simulink model "AM_passband"  (R2026a)
settings: Solver=VariableStepAuto  StopTime=1
model workspace (MAT data in the model file):
  FrameSize = 1000
  Fs = 100000
libraries: dspsrcs4 x3, dspfdesign x2, commchan3 x1
settings Model: Creator=ranja  LastModifiedBy=ranja

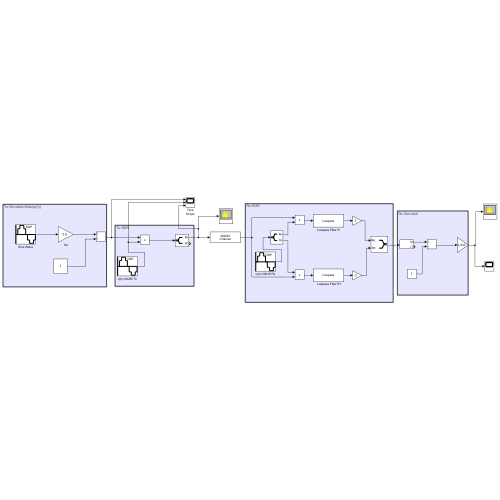
[thumbnail: Simulink's stored preview of the top-level diagram]
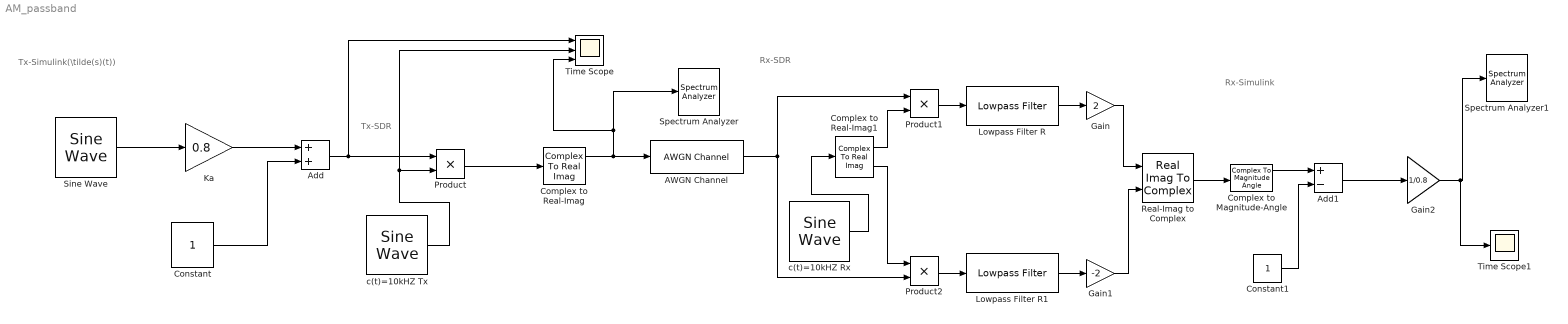
== system AM_passband ==
  note: Rx-Simulink
  note: Rx-SDR
  note: Tx-SDR
  note: Tx-Simulink(\tilde(s)(t))
  " Ka" : Gain  Gain=0.8
  AWGN Channel : commchan3/AWGN Channel  LegacyMode=off  NoiseMethod="Signal to noise ratio  (SNR)"  noiseMode="Signal to noise ratio  (SNR)"  EbNo=10  EsNo=10  SNR=10  BitsPerSymbol=1  SignalPower=1  SpecifySymbolPeriod=off  SamplesPerSymbol=1  SymbolPeriod=1  VarianceSource=Parameter  Variance=1  RandomStream=Global stream  Seed=67  SimulateUsing=Code generation
  Add : Sum
  Add1 : Sum  Inputs=+-
  Complex to Magnitude-Angle : ComplexToMagnitudeAngle
  Complex to Real-Imag : ComplexToRealImag
  Complex to Real-Imag1 : ComplexToRealImag
  Constant : Constant
  Constant1 : Constant
  Gain : Gain  Gain=2
  Gain1 : Gain  Gain=-2
  Gain2 : Gain  Gain=1/0.8
  Lowpass Filter R : dspfdesign/Lowpass Filter  FilterType=FIR  DesignForMinimumOrder=off  FilterOrder=50  PassbandFrequency=1100  StopbandFrequency=0.5442  PassbandRipple=0.1  StopbandAttenuation=80  SampleRateMode=Specify on dialog  SampleRate=Fs  SimulateUsing=Interpreted execution  roundingMode=Floor  coeffsDataTypeStr=fixdt(1,16)
  Lowpass Filter R1 : dspfdesign/Lowpass Filter  FilterType=FIR  DesignForMinimumOrder=off  FilterOrder=50  PassbandFrequency=1100  StopbandFrequency=0.5442  PassbandRipple=0.1  StopbandAttenuation=80  SampleRateMode=Specify on dialog  SampleRate=Fs  SimulateUsing=Interpreted execution  roundingMode=Floor  coeffsDataTypeStr=fixdt(1,16)
  Product : Product
  Product1 : Product
  Product2 : Product
  Real-Imag to Complex : RealImagToComplex
  Sine Wave : dspsrcs4/Sine Wave  Amplitude=1  Frequency=1000  Phase=0  SampleMode=Discrete  OutComplex=Real  CompMethod=Trigonometric fcn  TableSize=Speed  SampleTime=1/Fs  SamplesPerFrame=FrameSize  ResetState=Restart at time zero  OutputFrames=off  dataType=double  wordLen=16  udDataType=sfix(16)  fracBitsMode=Best precision  numFracBits=15  OutDataTypeStr=double  LastOutDataTypeStr=double
  Spectrum Analyzer : SpectrumAnalyzer  WindowPosition=[368.000000,182.000000,800.000000,500.000000,]  ScopeFrameLocation=window  WindowInvariantSamplesPerUpdate=on  Span=100000  StartFrequency=-50000  StopFrequency=50000  YLimits=[-83.7362 34.2546]
  Spectrum Analyzer1 : SpectrumAnalyzer  WindowPosition=[1.000000,49.000000,1536.000000,793.000000,]  ScopeFrameLocation=window  WindowInvariantSamplesPerUpdate=on  FrequencySpan=Span and center frequency  Span=50000  StartFrequency=-50000  StopFrequency=50000  YLimits=[-68.0974 28.8861]  SelectedToolstripTab=spectrumAnalyzerToolstrip.estimationTab
  Time Scope : Scope  NumInputPorts=3
      settings: TimeUnits=Metric (based on Time Span)  ActiveDisplayYMinimum=0.21609485710194476  ActiveDisplayYMaximum=1.7356972505215549  YLabel=Amplitude
  Time Scope1 : Scope
      settings: TimeUnits=Metric (based on Time Span)  ActiveDisplayYMinimum=-1.3427014205665166  ActiveDisplayYMaximum=1.6995374742641378  YLabel=Amplitude
  c(t)=10kHZ Rx : dspsrcs4/Sine Wave  Amplitude=1  Frequency=10000  Phase=0  SampleMode=Discrete  OutComplex=Complex  CompMethod=Trigonometric fcn  TableSize=Speed  SampleTime=1/Fs  SamplesPerFrame=FrameSize  ResetState=Restart at time zero  OutputFrames=off  dataType=double  wordLen=16  udDataType=sfix(16)  fracBitsMode=Best precision  numFracBits=15  OutDataTypeStr=double  LastOutDataTypeStr=double
  c(t)=10kHZ Tx : dspsrcs4/Sine Wave  Amplitude=1  Frequency=10000  Phase=0  SampleMode=Discrete  OutComplex=Complex  CompMethod=Trigonometric fcn  TableSize=Speed  SampleTime=1/Fs  SamplesPerFrame=FrameSize  ResetState=Restart at time zero  OutputFrames=off  dataType=double  wordLen=16  udDataType=sfix(16)  fracBitsMode=Best precision  numFracBits=15  OutDataTypeStr=double  LastOutDataTypeStr=double
  wires:
  Sine Wave/1 -> " Ka"/1
  " Ka"/1 -> Add/1
  Constant/1 -> Add/2
  Add/1 -> Time Scope/1, Product/1
  c(t)=10kHZ Tx/1 -> Time Scope/2, Product/2
  Product/1 -> Complex to Real-Imag/1
  Complex to Real-Imag/1 -> Time Scope/3, Spectrum Analyzer/1, AWGN Channel/1
  c(t)=10kHZ Rx/1 -> Complex to Real-Imag1/1
  AWGN Channel/1 -> Product2/2, Product1/1
  Complex to Real-Imag1/1 -> Product1/2
  Complex to Real-Imag1/2 -> Product2/1
  Product1/1 -> Lowpass Filter R/1
  Product2/1 -> Lowpass Filter R1/1
  Lowpass Filter R/1 -> Gain/1
  Lowpass Filter R1/1 -> Gain1/1
  Gain/1 -> Real-Imag to Complex/1
  Gain1/1 -> Real-Imag to Complex/2
  Real-Imag to Complex/1 -> Complex to Magnitude-Angle/1
  Complex to Magnitude-Angle/1 -> Add1/1
  Constant1/1 -> Add1/2
  Add1/1 -> Gain2/1
  Gain2/1 -> Time Scope1/1, Spectrum Analyzer1/1
